simulink model "sim_ekf_est_4para_variable_load"  (R2020b)
settings: Solver=ode1  StartTime=0.0  StopTime=150  FixedStep=0.01  RelTol=1e-3
settings Model: Creator=Admin  LastModifiedBy=ONLY-GOD

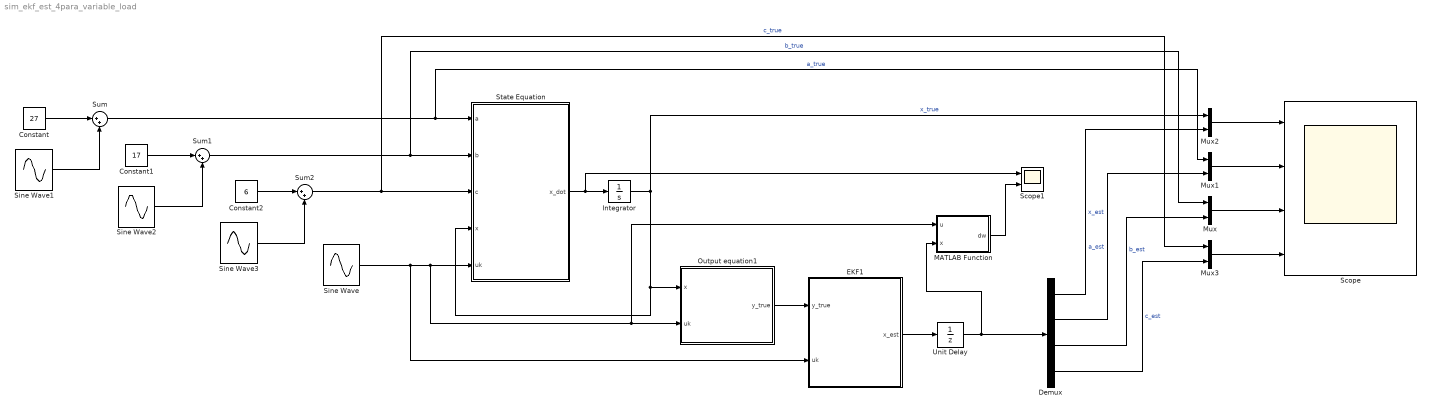
== system sim_ekf_est_4para_variable_load ==
  Constant : Constant  Value=27
  Constant1 : Constant  Value=17
  Constant2 : Constant  Value=6
  Demux : Demux
  EKF1 : MATLAB Function  TreatAsAtomicUnit=on
  Integrator : Integrator
  MATLAB Function : MATLAB Function  TreatAsAtomicUnit=on
  Mux{,1..3} (4 alike) : Mux  Inputs=2
  Output equation1 : MATLAB Function  TreatAsAtomicUnit=on
  Scope : Scope  NumInputPorts=4
  Scope1 : Scope  NumInputPorts=2
  Sine Wave : Sin  Amplitude=20  Frequency=2*pi*0.1  SampleTime=0
  Sine Wave1 : Sin  Amplitude=27*0.1  Frequency=2*pi*0.1  SampleTime=0
  Sine Wave2 : Sin  Amplitude=17*0.1  Frequency=2*pi/4  SampleTime=0
  Sine Wave3 : Sin  Amplitude=6*0.1  Frequency=2*pi*0.1  SampleTime=0
  State Equation : MATLAB Function  TreatAsAtomicUnit=on
  Sum : Sum  Inputs=|++
  Sum1 : Sum  Inputs=|++
  Sum2 : Sum  Inputs=|++
  Unit Delay : UnitDelay  InitialCondition=[0;0;0;0]  SampleTime=-1  HasFrameUpgradeWarning=on
  wires:
  Integrator/1 -> Mux2/1, Output equation1/1(x), State Equation/4(x)  "x_true"
  Sum/1 -> State Equation/1(a), Mux1/1  "a_true"
  Sum1/1 -> Mux/1, State Equation/2(b)  "b_true"
  Sine Wave/1 -> EKF1/2(uk), MATLAB Function/1(u), Output equation1/2(uk), State Equation/5(uk)
  Sum2/1 -> State Equation/3(c), Mux3/1  "c_true"
  State Equation/1(x_dot) -> Scope1/1, Integrator/1
  Constant/1 -> Sum/1
  Sine Wave1/1 -> Sum/2
  Constant1/1 -> Sum1/1
  Sine Wave2/1 -> Sum1/2
  Constant2/1 -> Sum2/1
  Sine Wave3/1 -> Sum2/2
  EKF1/1(x_est) -> Unit Delay/1
  Output equation1/1(y_true) -> EKF1/1(y_true)
  Unit Delay/1 -> MATLAB Function/2(x), Demux/1
  Mux2/1 -> Scope/1
  Mux1/1 -> Scope/2
  Mux/1 -> Scope/3
  Mux3/1 -> Scope/4
  Demux/4 -> Mux3/2  "c_est"
  Demux/3 -> Mux/2  "b_est"
  Demux/2 -> Mux1/2  "a_est"
  Demux/1 -> Mux2/2  "x_est"
  MATLAB Function/1(dw) -> Scope1/2

== matlab function sim_ekf_est_4para_variable_load/MATLAB Function ==
  data: u input; dw output; x input
function dw = fcn(u,x)

dw = -x(2)*x(1)+x(3)*u-x(4)*sign(x(1));

== matlab function sim_ekf_est_4para_variable_load/State Equation ==
  settings: updateMethod=DISCRETE
  data: a input; b input; c input; x input; uk input; x_dot output
function x_dot = state_eq(a,b,c,x,uk)
% x1 = W , x2 = a , x3 = b , x4 = c
x_dot = -a*x + b*uk - c*sign(x);

== matlab function sim_ekf_est_4para_variable_load/EKF1 ==
  settings: updateMethod=DISCRETE
  data: y_true input; uk input; x_est output
function x_est = ekf(y_true, uk)
Ts = 0.01;
persistent x_est_p P Qd_est R_est Qc_est;
if isempty(x_est_p)
    x_est_p = [0;0;0;0];
    P       = 1*diag([10,1,30,10]);
    Qc_est  = 1e-3*diag([1,10,100,10]);
    Qd_est  = Ts*Qc_est;
    R_est   = 0.01;
end
c  = [1 0 0 0];
D  = 0;
Ck = c;
Dk = D;

%Comput Kalman Gain and update predicted value
Wk    = P*Ck'/(Ck*P*Ck'+R_est);
y_est = Ck*x_est_p+Dk*uk;
x     = x_est_p+Wk*(y_true-y_est);

%Compute prediction at next time step
x_est = x+Ts*[-x(2)*x(1)+uk*x(3)-x(4)*sign(x(1));
                          0;
                          0;
                          0];

%Update error covariance matrices
P = P-Wk*Ck*P;

%Define Ak
Ak      = eye(4)+Ts*[-x(2) -x(1) uk -sign(x(1));
                 0     0    0      0;
                 0     0    0      0;
                 0     0    0      0];
P       = Ak*P*Ak'+Qd_est;
x_est_p = x_est;

== matlab function sim_ekf_est_4para_variable_load/Output equation1 ==
  settings: updateMethod=DISCRETE
  data: x input; uk input; y_true output
function y_true = output_eq(x,uk)
C = 1;
D = 0;
y_true = C*x+D*uk+sqrt(0.02)*randn;
